simulink model "S3_6"  (R2020b)
settings: Solver=VariableStepAuto  StartTime=0.0  StopTime=20  RelTol=1e-3
undefined symbols (not defined in the file or in its folder): DiscIntNeverNeededParam
libraries: simulink x1
settings Model: Creator=vicgd  LastModifiedBy=vicgd

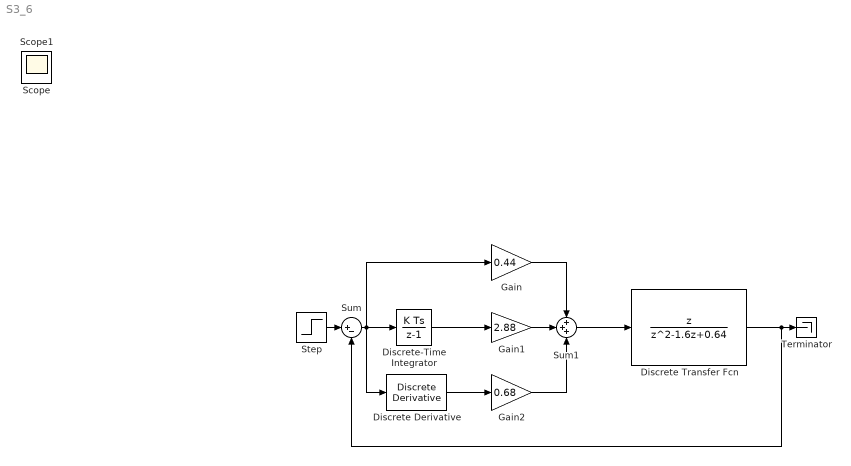
== system S3_6 ==
  Discrete Transfer Fcn : DiscreteTransferFcn  Numerator=[1 0]  Denominator=[1 -1.6 0.64]
  Discrete Derivative : simulink/Discrete/Discrete Derivative  gainval=1  ICPrevScaledInput=0.0  OutMin=[]  OutMax=[]  OutDataType=fixdt(1, 16)  OutScaling=2^-10  DoSatur=off
  Discrete-Time Integrator : DiscreteIntegrator  SampleTime=-1  ICPrevOutput=DiscIntNeverNeededParam  ICPrevScaledInput=DiscIntNeverNeededParam
  Gain : Gain  Gain=0.44
  Gain1 : Gain  Gain=2.88
  Gain2 : Gain  Gain=0.68
  Step : Step  SampleTime=1
  Sum : Sum  Inputs=|+-
  Sum1 : Sum  Inputs=+++
  Terminator : Terminator
  Scope : Scope
  Scope1 : Scope
  wires:
  Discrete Transfer Fcn/1 -> Terminator/1, Sum/2
  Step/1 -> Sum/1
  Sum/1 -> Gain/1, Discrete-Time Integrator/1, Discrete Derivative/1
  Discrete Derivative/1 -> Gain2/1
  Discrete-Time Integrator/1 -> Gain1/1
  Gain/1 -> Sum1/1
  Gain1/1 -> Sum1/2
  Gain2/1 -> Sum1/3
  Sum1/1 -> Discrete Transfer Fcn/1
